simulink model "MMS_ESC_LSQ"  (R2019b)
settings: Solver=ode3  StartTime=par.sym.TStart  StopTime=par.sym.TStop  FixedStep=par.sym.max_dt  MaxStep=par.sym.max_dt  RelTol=1e-3
undefined symbols (not defined in the file): a_K, B, b, k, K_0, K_init, k_K, m, N_buff, N_delay, par, Sat, T_tran, W_K, w_K, w_wav
libraries: simulink x1
settings Model: Creator=Vitù  LastModifiedBy=User
settings SolverCC: AutoInsertRateTranBlk=on
settings DataIOCC: SaveFormat=Array  SaveOutput=off  SignalLogging=off  DSMLogging=off  ReturnWorkspaceOutputs=off  TimeSaveName=TIME  OutputSaveName=Yout  OutputOption=SpecifiedOutputTimes  OutputTimes=[par.sym.TStart:par.sym.Outputdt:par.sym.TStop]
settings OptimizationCC: ExpressionDepthLimit=2147483647  LifeSpan=inf
settings DebuggingCC: UnderspecifiedInitializationDetection=Classic  MergeDetectMultiDrivingBlocksExec=none  SolverPrmCheckMsg=warning  AllowSymbolicDim=off  StateNameClashWarn=warning  SFUnexpectedBacktrackingDiag=warning  SFNoUnconditionalDefaultTransitionDiag=warning  SFExecutionAtInitializationDiag=none  ArithmeticOperatorsInVariantConditions=warning
settings HardwareCC: ProdBitPerPointer=32  ProdBitPerSizeT=32  ProdBitPerPtrDiffT=32  ProdLargestAtomicFloat=None  ProdIntDivRoundTo=Undefined  ProdEndianess=Unspecified  ProdWordSize=32  ProdHWDeviceType=32-bit Generic
settings ModelReferenceCC: PropagateSignalLabelsOutOfModel=off
settings SFSimCC: SimUseLocalCustomCode=off  CustomCodeUndefinedFunction=UseInterfaceOnly
settings RTWCC: GenCodeOnly=on  RTWUseLocalCustomCode=off
settings CodeAppCC: StateflowObjectComments=on
settings GRTTargetCC: TargetLangStandard=C89/C90 (ANSI)  GeneratePreprocessorConditionals=Disable all
settings ConfigComp: CovMetricSettings=dw  CovHtmlReporting=on  CovSaveCumulativeToWorkspaceVar=on  CovSaveSingleToWorkspaceVar=on  CovExternalEMLEnable=off  CovSFcnEnable=off
settings SimscapeCC: SimscapeNormalizeSystem=off
settings ConfigurationSet: Description=SimMechanics 2G

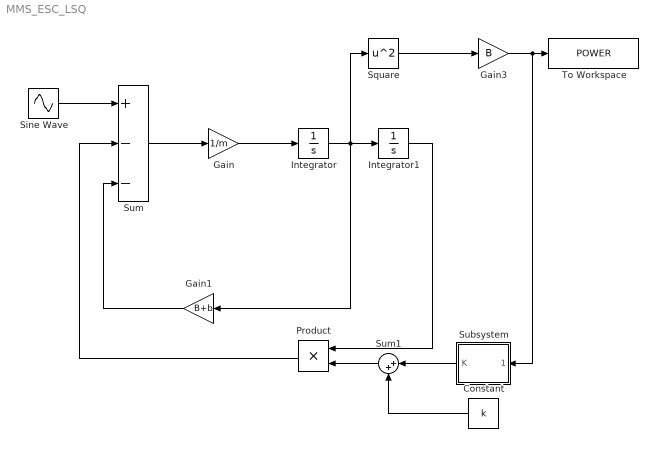
== system MMS_ESC_LSQ ==
  Constant : Constant  Value=k
  Gain : Gain  Gain=1/m
  Gain1 : Gain  Gain=B+b
  Gain3 : Gain  Gain=B
  Integrator : Integrator
  Integrator1 : Integrator
  Product : Product
  Sine Wave : Sin  Amplitude=par.H  Frequency=w_wav  SampleTime=0
  Square : Math  Operator=square  SignedPower=off  SaturateOnIntegerOverflow=on
  Subsystem : Subsystem
  Sum : Sum  Inputs=+--
  Sum1 : Sum  Inputs=|++
  To Workspace : ToWorkspace  VariableName=POWER  SampleTime=-1
  wires:
  Product/1 -> Sum/2
  Gain3/1 -> Subsystem/1(POWER), To Workspace/1
  Integrator/1 -> Square/1, Gain1/1, Integrator1/1
  Gain/1 -> Integrator/1
  Gain1/1 -> Sum/3
  Square/1 -> Gain3/1
  Sum/1 -> Gain/1
  Integrator1/1 -> Product/1
  Sine Wave/1 -> Sum/1
  Subsystem/1(K) -> Sum1/1
  Sum1/1 -> Product/2
  Constant/1 -> Sum1/2

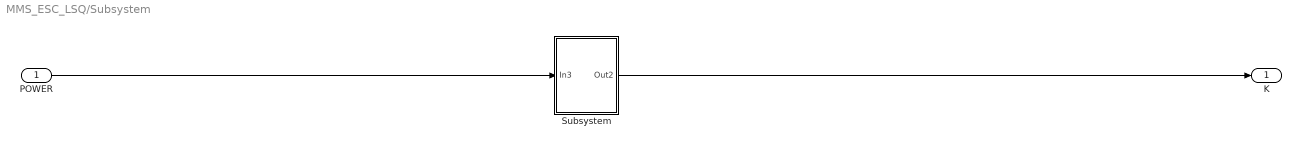
== system MMS_ESC_LSQ/Subsystem ==
  POWER : Inport
  Subsystem : Subsystem
  K : Outport
  wires:
  POWER/1 -> Subsystem/1(In3)
  Subsystem/1(Out2) -> K/1

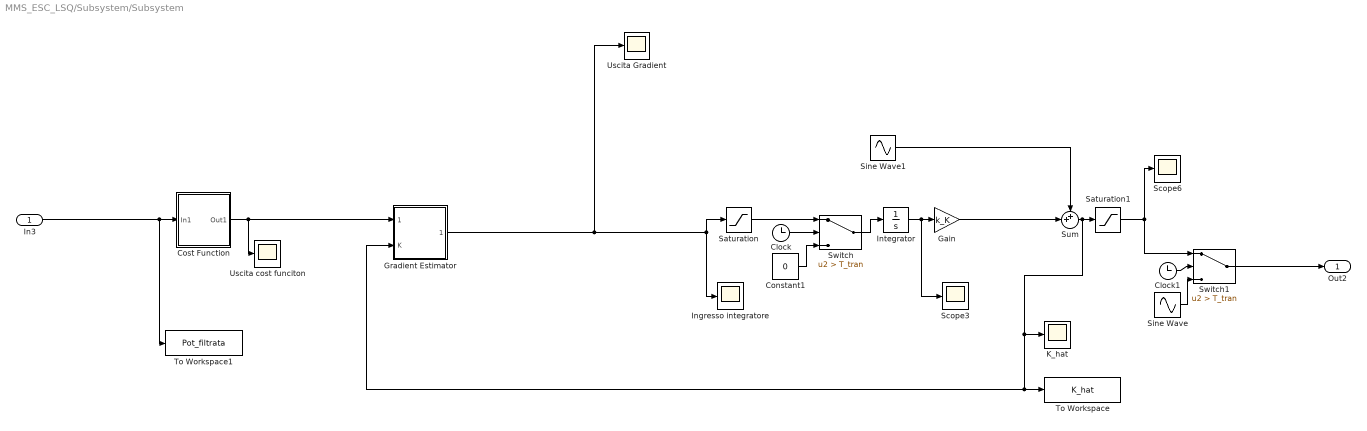
== system MMS_ESC_LSQ/Subsystem/Subsystem ==
  In3 : Inport
  Clock : Clock
  Clock1 : Clock
  Constant1 : Constant  Value=0
  Cost Function : Subsystem
  Gain : Gain  Gain=k_K
  Gradient Estimator : Subsystem
  Ingresso integratore : Scope
  Integrator : Integrator  InitialCondition=K_init
  K_hat : Scope
  Saturation : Saturate  UpperLimit=Sat  LowerLimit=-Sat
  Saturation1 : Saturate  UpperLimit=inf  LowerLimit=-k
  Scope3 : Scope
  Scope6 : Scope
  Sine Wave : Sin  Amplitude=50  Bias=K_0  Frequency=w_wav  SampleTime=0
  Sine Wave1 : Sin  Amplitude=a_K  Frequency=w_K  SampleTime=0
  Sum : Sum  Inputs=++|
  Switch : Switch  Criteria=u2 > Threshold  Threshold=T_tran
  Switch1 : Switch  Criteria=u2 > Threshold  Threshold=T_tran
  To Workspace : ToWorkspace  VariableName=K_hat  SampleTime=-1
  To Workspace1 : ToWorkspace  VariableName=Pot_filtrata  SampleTime=-1
  Uscita Gradient : Scope
  Uscita cost funciton : Scope
  Out2 : Outport
  wires:
  Constant1/1 -> Switch/3
  Gradient Estimator/1(Derivative) -> Uscita Gradient/1, Saturation/1, Ingresso integratore/1
  Gain/1 -> Sum/2
  Switch1/1 -> Out2/1
  Switch/1 -> Integrator/1
  Clock/1 -> Switch/2
  Saturation/1 -> Switch/1
  Clock1/1 -> Switch1/2
  Integrator/1 -> Scope3/1, Gain/1
  Cost Function/1(Out1) -> Uscita cost funciton/1, Gradient Estimator/1(Performance Function)
  In3/1 -> To Workspace1/1, Cost Function/1(In1)
  Sum/1 -> Gradient Estimator/2(K), To Workspace/1, K_hat/1, Saturation1/1
  Sine Wave/1 -> Switch1/3
  Sine Wave1/1 -> Sum/1
  Saturation1/1 -> Switch1/1, Scope6/1

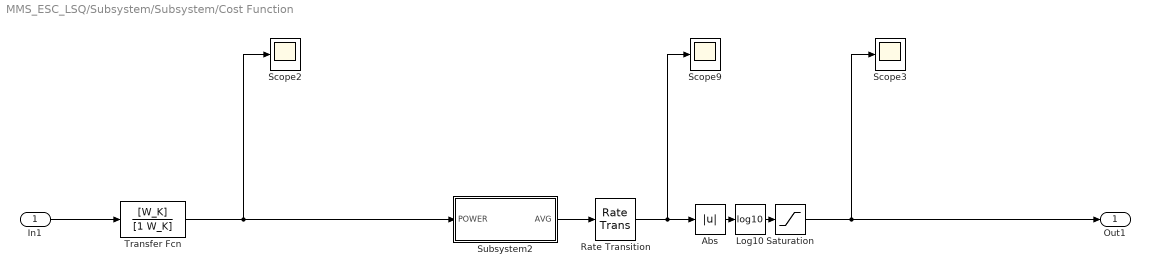
== system MMS_ESC_LSQ/Subsystem/Subsystem/Cost Function ==
  In1 : Inport
  Abs : Abs
  Log10 : Math  Operator=log10  SignedPower=off  SaturateOnIntegerOverflow=on
  Rate Transition : RateTransition
  Saturation : Saturate  UpperLimit=inf  LowerLimit=-40
  Scope2 : Scope
  Scope3 : Scope
  Scope9 : Scope
  Subsystem2 : Subsystem
  Transfer Fcn : TransferFcn  Numerator=[W_K]  Denominator=[1 W_K]
  Out1 : Outport
  wires:
  Subsystem2/1(AVG) -> Rate Transition/1
  Rate Transition/1 -> Abs/1, Scope9/1
  In1/1 -> Transfer Fcn/1
  Transfer Fcn/1 -> Subsystem2/1(POWER), Scope2/1
  Abs/1 -> Log10/1
  Log10/1 -> Saturation/1
  Saturation/1 -> Out1/1, Scope3/1

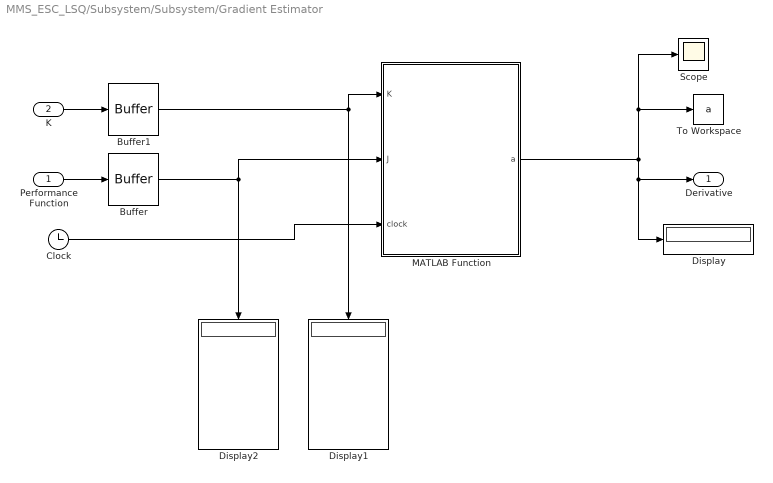
== system MMS_ESC_LSQ/Subsystem/Subsystem/Gradient Estimator ==
  Performance Function : Inport  SampleTime=1
  K : Inport  Port=2  SampleTime=1
  Buffer : Buffer  N=N_buff  V=N_buff-1  OutputFrames=off
  Buffer1 : Buffer  N=N_buff  V=N_buff-1  OutputFrames=off
  Clock : Clock
  Display : Display
  Display1 : Display
  Display2 : Display
  MATLAB Function : MATLAB Function  TreatAsAtomicUnit=on
  Scope : Scope
  To Workspace : ToWorkspace  VariableName=a  SaveFormat=Timeseries  SampleTime=-1
  Derivative : Outport
  wires:
  Buffer1/1 -> Display1/1, MATLAB Function/1(K)
  K/1 -> Buffer1/1
  Performance Function/1 -> Buffer/1
  Buffer/1 -> MATLAB Function/2(J), Display2/1
  MATLAB Function/1(a) -> To Workspace/1, Scope/1, Display/1, Derivative/1
  Clock/1 -> MATLAB Function/3(clock)

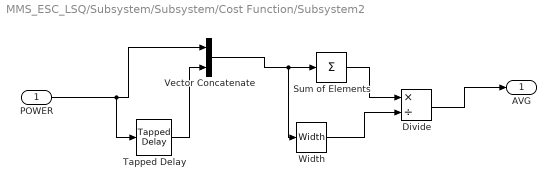
== system MMS_ESC_LSQ/Subsystem/Subsystem/Cost Function/Subsystem2 ==
  POWER : Inport
  Divide : Product  Inputs=*/
  Sum of Elements : Sum  Inputs=+
  Tapped Delay : simulink/Discrete/Tapped Delay  vinit=0  samptime=-1  NumDelays=N_delay  DelayOrder=Oldest  includeCurrent=off
  Vector Concatenate : Concatenate
  Width : Width
  AVG : Outport
  wires:
  POWER/1 -> Tapped Delay/1, Vector Concatenate/1
  Tapped Delay/1 -> Vector Concatenate/2
  Vector Concatenate/1 -> Width/1, Sum of Elements/1
  Sum of Elements/1 -> Divide/1
  Width/1 -> Divide/2
  Divide/1 -> AVG/1

== matlab function MMS_ESC_LSQ/Subsystem/Subsystem/Gradient Estimator/MATLAB Function ==
  data: K input; J input; clock input; a output

function a = LSQ(K,J,clock)
if clock > 25
    p = polyfit(K,J,1);
    a = p(1);
%    l = max( [-(log(abs(v))) 9]);
%    l = -log(abs(v));
%     if l<0
%         l=0;
%     end
%   v = v*10^(l);
%    s = sign(v);
%    v=abs(v);
%    v = min([v 0.5]);
%    a = R*s;
else
    a = 0;
    %l=0;
end

end
